simulink model "Bands3"  (R2018a)
settings: Solver=VariableStepAuto  StartTime=0.0  StopTime=0.01  RelTol=1e-3
undefined symbols (not defined in the file): fdesignblkfcn, G1, G2, G3, gcbh, get, T
libraries: dspsrcs4 x1, dspxfrm3 x1, dspobslib x1
settings Model: Creator=Daniel  LastModifiedBy=Daniel

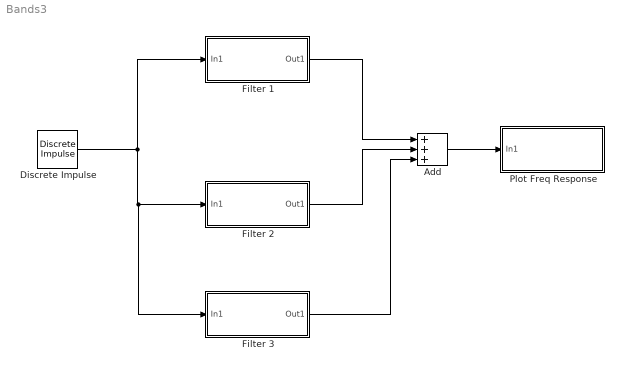
== system Bands3 ==
  Add : Sum  Inputs=+++
  Discrete Impulse : dspsrcs4/Discrete  Impulse  Delay=0  SampleTime=T  FrameSample=128  OutputFrames=off  dataType=double  isSigned=on  wordLen=16  udDataType=sfix(16)  fracBitsMode=Best precision  numFracBits=15  OutDataTypeStr=double  LastOutDataTypeStr=double
  Filter 1 : Subsystem
  Filter 2 : Subsystem
  Filter 3 : Subsystem
  Plot Freq Response : Subsystem
  wires:
  Discrete Impulse/1 -> Filter 3/1(In1), Filter 2/1(In1), Filter 1/1(In1)
  Add/1 -> Plot Freq Response/1(In1)
  Filter 1/1(Out1) -> Add/1
  Filter 2/1(Out1) -> Add/2
  Filter 3/1(Out1) -> Add/3

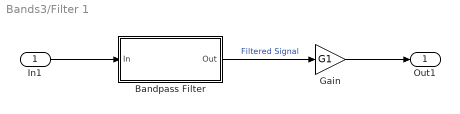
== system Bands3/Filter 1 ==
  In1 : Inport
  Bandpass Filter : Subsystem  DialogController=fdesignblkfcn  InitFcn=fdesignblkfcn(gcbh, {'InitFcn'});  mask(Bandpass Filter){}
      mask help: Design a bandpass filter
      settings: CopyFcn=fdesignblkfcn(gcbh, {'CopyFcn'});
      mask Help: helpview(mapfilelocation('dsp'), 'dspbandpassfilter');
      mask Display: disp('Bandpass');
  Gain : Gain  Gain=G1
  Out1 : Outport
  wires:
  Bandpass Filter/1(Out) -> Gain/1  "Filtered Signal"
  In1/1 -> Bandpass Filter/1(In)
  Gain/1 -> Out1/1

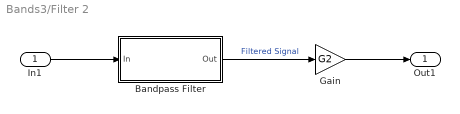
== system Bands3/Filter 2 ==
  In1 : Inport
  Bandpass Filter : Subsystem  DialogController=fdesignblkfcn  InitFcn=fdesignblkfcn(gcbh, {'InitFcn'});  mask(Bandpass Filter){}
      mask help: Design a bandpass filter
      settings: CopyFcn=fdesignblkfcn(gcbh, {'CopyFcn'});
      mask Help: helpview(mapfilelocation('dsp'), 'dspbandpassfilter');
      mask Display: disp('Bandpass');
  Gain : Gain  Gain=G2
  Out1 : Outport
  wires:
  Bandpass Filter/1(Out) -> Gain/1  "Filtered Signal"
  In1/1 -> Bandpass Filter/1(In)
  Gain/1 -> Out1/1

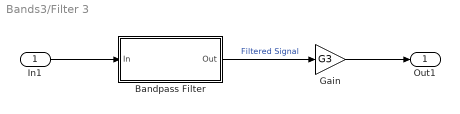
== system Bands3/Filter 3 ==
  In1 : Inport
  Bandpass Filter : Subsystem  DialogController=fdesignblkfcn  InitFcn=fdesignblkfcn(gcbh, {'InitFcn'});  mask(Bandpass Filter){}
      mask help: Design a bandpass filter
      settings: CopyFcn=fdesignblkfcn(gcbh, {'CopyFcn'});
      mask Help: helpview(mapfilelocation('dsp'), 'dspbandpassfilter');
      mask Display: disp('Bandpass');
  Gain : Gain  Gain=G3
  Out1 : Outport
  wires:
  Bandpass Filter/1(Out) -> Gain/1  "Filtered Signal"
  In1/1 -> Bandpass Filter/1(In)
  Gain/1 -> Out1/1

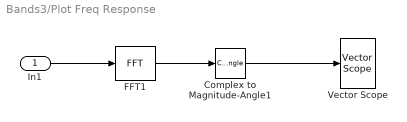
== system Bands3/Plot Freq Response ==
  In1 : Inport
  Complex to Magnitude-Angle1 : ComplexToMagnitudeAngle  Output=Magnitude
  FFT1 : dspxfrm3/FFT  FFTImplementation=Auto  CompMethod=Table lookup  TableOpt=NEW  TableOptActive=Speed  BitRevOrder=off  Normalize=off  InheritFFTLength=on  FFTLength=64  WrapInput=on  roundingMode=Floor  overflowMode=off  firstCoeffDataTypeStr=Inherit: Same word length as input  firstCoeffLastDataTypeStr=Inherit: Same word length as input  outputMin=[]  outputMax=[]
  Vector Scope : dspobslib/Vector Scope  ScopeProperties=off  Domain=Frequency  HorizSpan=1  DisplayProperties=off  AxisGrid=on  Memory=off  FrameNumber=off  AxisLegend=off  AxisZoom=off  OpenScopeAtSimStart=on  OpenScopeImmediately=off  FigPos=get(0,'defaultfigureposition')  AxisProperties=on  XUnits=Hertz  XRange=[0...Fs/2]  InheritXIncr=on  XIncr=1  XLabel=Samples  XLimit=Auto  XMin=0  XMax=1  XStart=0  YUnits=dB  YLabel=|Magnitude (dB)|  LineProperties=off  XAxisParamsVer=6.9
      settings: SourceProductName=DSP System Toolbox  SourceProductBaseCode=DS  YMin=0.0723692553519949  YMax=69.3188381671759
  wires:
  In1/1 -> FFT1/1
  FFT1/1 -> Complex to Magnitude-Angle1/1
  Complex to Magnitude-Angle1/1 -> Vector Scope/1

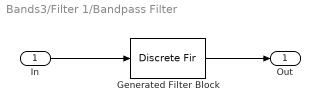
== system Bands3/Filter 1/Bandpass Filter ==
  In : Inport
  Generated Filter Block : DiscreteFir  Tag=BlockMethodSubSystem  Coefficients=[-6.40576144934966193e-06 -3.97953670873177584e-05 -0.000144137650217380961 -0.000383800486190155089 -0.000817210421981588416 -0.00144442932314671306 -0.00214735235061815338 -0.00266286690640505893 -0.00263294689862399525 -0.00174654039451016953 6.93454980413866226e-05 0.0025079221852439583 0.00490023482119538063 0.00644130197387373336 0.00655667000311531672 0.0052307229511706077 0.00309362126395213875 0.00116673431577386864 0.000358915481620498218 0.000977521237260041984 0.00254836387185212922 0.00408194937610235377 0.00465550554904706725 0.00396703160553122346 0.00251035403808889642 0.00124625803940191606 0.000971434274142956569 0.00179731301558658067 0.00309026300151621315 0.00391818842080219037 0.00369858428573058068 0.00259626774651279752 0.00138939911212525541 0.000899274950534003107 0.00139551031110889709 0.00240984656229591577 0.0030946597147498622 0.00285930992515541233 0.00180824282091297632 0.000651312769417266364 0.000155132883116135685 0.00055493140049561805 0.00137904290044887933 0.00182190248030878171 0.00137591825026365817 0.000228349084653821339 -0.000889647122507301207 -0.00128456211020466088 -0.000852862911503151624 -0.000163235324001641724 4.18646822138339452e-07 -0.000728131146705390917 -0.00199825967930350804 -0.00302297567760601276 -0.00321748260841813816 -0.00267903510737666373 -0.00211295854537262452 -0.00225738586678620899 -0.00327256296197019026 -0.00459854618067659371 -0.00540771026444777404 -0.00528802838358975041 -0.00459345388086216874 -0.00416216223701273459 -0.00462377036847594434 -0.00586559902268643345 -0.00710923104289114521 -0.00754844825884629523 -0.00702668665331728642 -0.00618453976387646053 -0.00593830323370301769 -0.00671097773610545949 -0.00805878118477507815 -0.00902114784188043708 -0.00891963853291183675 -0.0079419408108293895 -0.00700817723953940479 -0.00700994420116827187 -0.00804883251651217387 -0.0093227818329443303 -0.00977912137442263872 -0.00900387428505758196 -0.00759677215868335368 -0.00669363795363312787 -0.00701370567982918976 -0.00822902196139210437 -0.00920691165021869998 -0.00895010834930162757 -0.00745565042547421605 -0.00575403088988683548 -0.00506433772551448391 -0.00575611016767026487 -0.00700064113535321317 -0.00743709966997422971 -0.0063208611919999113 -0.00418701611938208582 -0.00244058376406157667 -0.00218360301464723102 -0.00325696419168262224 -0.00432889685252003768 -0.00399537071090265341 -0.00198628937933848816 0.000555807305062370723 0.00200140298389937191 0.00161578964150893697 0.000225987076418367378 -0.000430263671310224705 0.000833719393189015327 0.00360704612833227757 0.0061684884550191315 0.00691456873172264716 0.00574462117577661385 0.0042071809637693712 0.00423031324569863275 0.00647200446559058687 0.00969752191187244796 0.0117637112870944763 0.0114283526644724433 0.00945798106402909178 0.00804848512766443043 0.00898716390757738244 0.0120894716893311278 0.0152719743477611556 0.0162686295262881517 0.0145787329543523199 0.0119738485068503261 0.0110632515100516377 0.0130728721556965383 0.0167227649975076401 0.0192216360330200314 0.0186122330086842536 0.0154998061429673477 0.0126415138185526129 0.0126559242458025752 0.0157490315970162803 0.0194247891479758517 0.0205212417808085523 0.0179170804912010748 0.0135969997082004117 0.0110770938941794628 0.012429702469166656 0.016417931911488489 0.0194086367432017223 0.0184066618804281587 0.0136842174605042999 0.00870674372852131562 0.00728566234734476584 0.0102878852489942281 0.0147331460745012827 0.0161841836591450905 0.0125264834220616961 0.00593048682077353725 0.00119685413102984801 0.0017270344872468181 0.0064887066933950405 0.0106666277702681458 0.00964000113177999191 0.00301951793584741149 -0.00476136667546827978 -0.00801757145812169274 -0.00468938245289579701 0.00163749107944401043 0.00450380399818216259 3.13890464266591146e-05 -0.00951509161729160828 -0.0172861288360418967 -0.0175134761533925661 -0.0106306266803574724 -0.00334539439545458294 -0.00323457841834334011 -0.0121669776820483196 ...(+5167 chars)]  InputProcessing=Columns as channels (frame based)
  Out : Outport
  wires:
  In/1 -> Generated Filter Block/1
  Generated Filter Block/1 -> Out/1

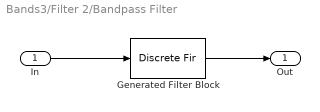
== system Bands3/Filter 2/Bandpass Filter ==
  In : Inport
  Generated Filter Block : DiscreteFir  Tag=BlockMethodSubSystem  Coefficients=[1.04348777191739433e-06 4.84326526690635391e-06 2.38197249221212201e-06 -2.35730568787196631e-05 -3.92046239602916778e-05 4.63373576906772283e-05 0.000166784820983319638 5.86828120487577722e-06 -0.000419688376950591926 -0.000307280437718730455 0.000694964922637293018 0.00103971419433206342 -0.000670834323369947066 -0.00217194334583996123 -7.72088565411671325e-05 0.00326756185482119949 0.00171699329596791705 -0.00359408048603206826 -0.00379778270085183185 0.00262875311255520144 0.00530117389286513356 -0.000635653118675858116 -0.00527615241575909999 -0.00126796997885316918 0.00365254722677240285 0.00182581097007843639 -0.00147406774645636863 -0.00066421675357351427 0.000168978923952104734 -0.00130492995865182961 -0.000379113395588064354 0.00259055002388848456 0.00141315488501136933 -0.00238489241344082151 -0.00190181739267116087 0.00121341916948340418 0.00108046610041277118 -0.000337846139618237426 0.000529196852115729438 0.000500429379813499922 -0.00168951432129683921 -0.00125490595900065965 0.00166689131012572674 0.00151615680856598462 -0.000869674581036881012 -0.000713984021226201 0.000313333555797200422 -0.000640209784151132355 -0.000533311930442181706 0.00150570919905014316 0.00108056097809560749 -0.00135825058904408638 -0.00107229430578221758 0.000648356733472345249 0.000174773742126788762 -0.000246626220516891104 0.00101239068635332156 0.000495044279146987466 -0.00155562834175254259 -0.000864210138755500167 0.00113920133310327766 0.000576108421475629551 -0.000367762815672993606 0.000466812342168897751 8.02009789329044087e-05 -0.00147064860000837108 -0.000398264026694880743 0.00155510499624480938 0.000586159905186488858 -0.00073326455529222471 4.72066947202601486e-05 -7.58862678444736086e-05 -0.00120369166718514936 0.000111104411520643488 0.00179347319491862276 0.000303773504431839201 -0.0011771735665706811 -0.000162706044442818956 -6.26477060013774599e-06 -0.000868770856363788304 0.000549088689737188356 0.00184143238325738617 -0.000163794874201824195 -0.0015824858613062839 -0.000145540896929906641 0.000214873756412053599 -0.000555426438079929569 0.000870142703780668689 0.00172891563680828224 -0.00072541526115845877 -0.00188005692033745356 7.45841313922558836e-05 0.000506608339207213288 -0.000315788283310417667 0.00107744328685374256 0.00149629927454698278 -0.00132315592271180964 -0.00203825307460487942 0.000462829543986070162 0.000804504830189103491 -0.000174258436810440165 0.00119287500999880141 0.00117915463067945784 -0.00192375119270570189 -0.00204860786184682441 0.000984759114910285479 0.00106821369529383047 -0.000134250966626290523 0.0012338130230592991 0.000794973690969484029 -0.00250167493410944708 -0.00190032153999456486 0.00160737371730785422 0.00126165971563733091 -0.000189755654587908239 0.00121958858306160677 0.000351855758743206866 -0.00303875104655445269 -0.00158155704159222547 0.00230065735445784524 0.00135138970026576631 -0.000330413278732329585 0.00117247418561423639 -0.000145470047162505754 -0.00352607350237420323 -0.00108733948553928531 0.00304157563546546056 0.00132082601372412686 -0.000542353342711128007 0.00109686426358235789 -0.000706124299709691775 -0.00394529663795911353 -0.00039628380319971045 0.00380911685120182255 0.00114342538098309858 -0.000820853629403293884 0.000996885637204027696 -0.00133033432035980625 -0.00427155320695593674 0.000507992342927492905 0.00457744561812258467 0.000797782587160095961 -0.00116158369918634629 0.000864032172920594548 -0.00201837006692902506 -0.0044590636011805785 0.00165110389494929925 0.00530118481210609983 0.000243490701981410488 -0.00155326129845871803 0.000708874484775483173 -0.00276371817489494669 -0.00447217664741842574 0.00304607124748028152 0.00593719107569575834 -0.000546287394235077102 -0.00198444053016171972 0.000524256891578901924 -0.00356432587977688299 -0.0042527031378769807 0.00472215562406726012 0.00642609827458878822 -0.00162438302608463323 -0.00244686921158402109 0.000322577102499549265 -0.00439793748642968232 -0.00374236030925391818 ...(+6792 chars)]  InputProcessing=Columns as channels (frame based)
  Out : Outport
  wires:
  In/1 -> Generated Filter Block/1
  Generated Filter Block/1 -> Out/1

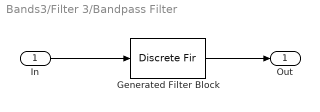
== system Bands3/Filter 3/Bandpass Filter ==
  In : Inport
  Generated Filter Block : DiscreteFir  Tag=BlockMethodSubSystem  Coefficients=[-1.13271540224336584e-06 6.14791156317734726e-06 -1.40623539368769451e-05 7.95223966381155355e-06 4.6031588785368761e-05 -0.00015941519188899435 0.000252074222717128295 -0.000143996176910986587 -0.000287531431111739402 0.000846846505916988047 -0.000961026265052958447 0.000110823057187895972 0.00144983376780560055 -0.00246215367464341006 0.00155361711565275254 0.00123209410232891442 -0.00384180514452992384 0.00368949748978298535 -0.000246666932052534097 -0.00388867254586983471 0.00505724273816263604 -0.0020902115886934072 -0.0023376584775576725 0.00428475170658055259 -0.00249734316786279827 -0.000563101102271991753 0.0017367606292007069 -0.000667615513389995864 -0.000300474658138253378 -0.000521040645282471295 0.00192391667388495165 -0.0015232488432748801 -0.00089021810056812286 0.00284037976000807869 -0.00222462682357086943 -7.11634126829384367e-05 0.00142345287353296815 -0.000846803302820994656 -3.02892165199026008e-05 -0.000448188159478018653 0.00153724080393215896 -0.00121583739773537154 -0.000782120027257146274 0.00236674616364964101 -0.00181646425346023311 2.13708609239232469e-05 0.000861560345594581094 -0.000359303443040995599 4.85211462058431528e-05 -0.000948562676423492322 0.00185009971397083169 -0.00106186914230885373 -0.000987729429119682621 0.00214367398386300844 -0.00139812041018430805 0.00011095588934543353 0.000117775252989370016 0.000281881580441139482 0.000228975270274811181 -0.0016627852489978839 0.00221075723805871319 -0.000826637788696739611 -0.00113641388989244203 0.00171452706359642715 -0.000942390326951553052 0.000471018553061746 -0.000883342319074918248 0.000838366807700328064 0.000652642427043081822 -0.00234497079952758003 0.00227629952503578814 -0.00052632646323728092 -0.000901378878628373821 0.000912924174237498957 -0.000628246269628046508 0.00126720237213670951 -0.00197606335412217268 0.00105450705615711942 0.00123002894646808271 -0.00262983845764482808 0.00191110310553704323 -0.000432360576612660628 -3.75075074260689553e-05 -0.000102628729104970172 -0.000739480875242112768 0.00239986796737151663 -0.0027599339551273752 0.000824310742826214141 0.00157650008225486003 -0.00218637210373004215 0.00131323636469653855 -0.000935538794486633681 0.00139519543795135238 -0.000887503877708851877 -0.00139209210646444571 0.0034019752659141156 -0.00283747479499889613 0.000414039601421141293 0.00115877753587779217 -0.0010239536099508229 0.00100350415017479264 -0.00221547084739347677 0.00288670583874843728 -0.000991744445394369088 -0.00225066079232610168 0.00360425915132886812 -0.00219167581326224978 0.000464765770566130827 -0.000309074073600793323 0.000321002839569973955 0.00149672761333629473 -0.00389528827178116854 0.00366703766818096298 -0.000414070557819423029 -0.00251749466759616835 0.00260919373508878465 -0.00142128756793623648 0.00161099702042936986 -0.00244990876526824481 0.000995041271791271891 0.00277526799058398343 -0.00502958187899788401 0.00325981938303992243 0.000129400478224647682 -0.00139073956638678079 0.000784687541656671613 -0.00149048483838972357 0.00385479100645525971 -0.00420621327008135516 0.000479662113242509665 0.0039734518059129139 -0.00464852601903813223 0.0020701200607458831 -0.00050243662986839755 0.00119105080055119752 -0.000698969002185086227 -0.00297474877325812218 0.00618984893945144672 -0.00445882193844929827 -0.000734929156438415983 0.00371588991937895794 -0.00261040929408213988 0.00141416867677374982 -0.00300148080261820535 0.00413359314367464734 -0.000612250033561987663 -0.00527578795668634873 0.00702426892294963356 -0.00306244693590965351 -0.00108895436698977434 0.00115303674936954978 -0.000145925646117966594 0.00271633948586445751 -0.00670411355278137215 0.00561675012726307096 0.0012092416184784926 -0.00657733627936195504 0.00533692841467056037 -0.00140473901911997785 0.00107808012497162954 -0.00301054949292166047 0.000702816723750079387 0.00614556850235521701 -0.00952612367088850366 0.00449376209873146842 0.00310844068282146004 -0.00489454003524128402 0.00191482307789394256 ...(+6742 chars)]  InputProcessing=Columns as channels (frame based)
  Out : Outport
  wires:
  In/1 -> Generated Filter Block/1
  Generated Filter Block/1 -> Out/1
